simulink model "a_1_Controllo_on_off_automa"  (R2019a)
settings: Solver=VariableStepAuto  StartTime=0.0  StopTime=50  RelTol=1e-3
values from neighbouring files (symbols this model uses):
  K = 0.5    [a.m]
  R = 0.5    [a.m]
settings Model: Creator=Samuele  LastModifiedBy=Samuele

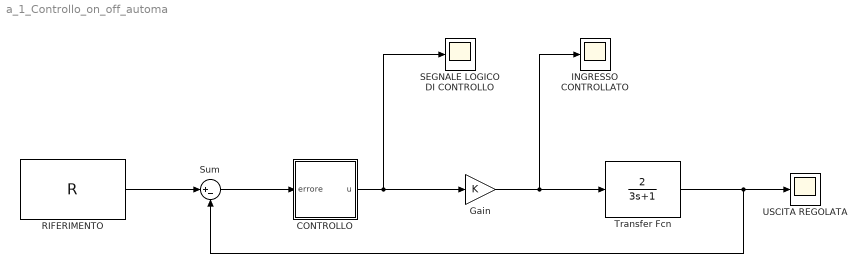
== system a_1_Controllo_on_off_automa ==
  CONTROLLO : Stateflow chart  BlockKeywords=__PRM__SERIALIZED__DATA__:Stateflow Chart,Stateflow Diagram  TreatAsAtomicUnit=on
  Gain : Gain  Gain=K
  INGRESSO CONTROLLATO : Scope
  RIFERIMENTO : Constant  Value=R
  SEGNALE LOGICO DI CONTROLLO : Scope
  Sum : Sum  Inputs=|+-
  Transfer Fcn : TransferFcn  Numerator=2  Denominator=[3 1]
  USCITA REGOLATA : Scope
  wires:
  RIFERIMENTO/1 -> Sum/1
  Sum/1 -> CONTROLLO/1(errore)
  Transfer Fcn/1 -> Sum/2, USCITA REGOLATA/1
  CONTROLLO/1(u) -> SEGNALE LOGICO DI CONTROLLO/1, Gain/1
  Gain/1 -> INGRESSO CONTROLLATO/1, Transfer Fcn/1

== stateflow chart a_1_Controllo_on_off_automa/CONTROLLO ==
  settings: updateMethod=CONTINUOUS
  state ON
    entry:
    u=1;
  state OFF
    entry:
    u=0;
  (default) -> ON
  OFF -> ON : [errore >= epsilon]
  ON -> OFF : [errore <= -epsilon]
  data: epsilon parameter; errore input; u output
  data u settings: updateMethod=SF_CONTINUOUS_TIME_DATA
